simulink library "Lib_Piccolo"  (R2018b)
settings: Solver=VariableStepAuto  StartTime=0.0  StopTime=10.0  RelTol=1e-3
values from neighbouring files (symbols this model uses):
  AccelErrInt2Brakes = 0.15    [SimulationControlConfig16P.m]    (also in SimulationControlConfig16P_F0.m; SimulationControlConfig16P_F2.m; SimulationControlConfig16P_LEGACY.m; SimulationControlConfigTAILLESS.m = 0.2)
  AileronMax = 25    [SimulationControlConfig16P.m]    (also in SimulationControlConfig16P_F0.m; SimulationControlConfig16P_F2.m; SimulationControlConfig16P_LEGACY.m; SimulationControlConfigTAILLESS.m)
  AileronPower = 0.00268    [SimulationControlConfig16P.m]    (also in SimulationControlConfig16P_F0.m; SimulationControlConfig16P_F2.m; SimulationControlConfig16P_LEGACY.m; SimulationControlConfigTAILLESS.m = 0.002266)
  AileronSurfaceMax = 45    [SimulationControlConfig16P.m]    (also in SimulationControlConfig16P_F0.m; SimulationControlConfig16P_F2.m; SimulationControlConfig16P_LEGACY.m; SimulationControlConfigTAILLESS_CGAFT_F0.m = 25)
  AileronTrim = 0    [SimulationControlConfig16P.m]    (also in SimulationControlConfig16P_F0.m; SimulationControlConfig16P_F2.m; SimulationControlConfig16P_LEGACY.m; SimulationControlConfigTAILLESS.m)
  Alt = 1000 + TerrainHeight    [SimulationStateConfig.m]
  AltCruise_m = Alt * 0.3048    [SimulationControlConfig16P.m]    (also in SimulationControlConfig16P_F2.m; SimulationControlConfigTAILLESS.m = Alt/3.28084; SimulationControlConfigTAILLESS_CGAFT_F0.m = 640; SimulationControlConfigTAILLESS_CGFWD_F0.m = 640)
  AltitudeRate2PitchCmdIntegratorInit = 0.1    [SimulationControlPre.m]
  AltMax = 10000    [SimulationControlConfig16P.m]    (also in SimulationControlConfig16P_F0.m; SimulationControlConfig16P_F2.m; SimulationControlConfig16P_LEGACY.m; SimulationControlConfigTAILLESS.m)
  AltMaxAccel = 2.5    [SimulationControlConfig16P.m]    (also in SimulationControlConfig16P_F0.m = 2; SimulationControlConfig16P_F2.m = 2; SimulationControlConfig16P_LEGACY.m = 0.9; SimulationControlConfigTAILLESS.m = 2)
  AltMin = 0    [SimulationControlConfig16P.m]    (also in SimulationControlConfig16P_F0.m; SimulationControlConfig16P_F2.m; SimulationControlConfig16P_LEGACY.m; SimulationControlConfigTAILLESS.m)
  AltRateCmd2Pitch = 0.26    [SimulationControlConfig16P.m]    (also in SimulationControlConfig16P_F0.m = 0.35; SimulationControlConfig16P_F2.m = 0.35; SimulationControlConfig16P_LEGACY.m = 0.6; SimulationControlConfigTAILLESS.m = 0.9)
  AltRateError2Pitch = 0.34    [SimulationControlConfig16P.m]    (also in SimulationControlConfig16P_F0.m = 0.61; SimulationControlConfig16P_F2.m = 0.61; SimulationControlConfig16P_LEGACY.m = 0.4; SimulationControlConfigTAILLESS.m = 0.3)
  AltRateErrorInt2Pitch = 0.61    [SimulationControlConfig16P.m]    (also in SimulationControlConfig16P_F0.m = 0.28; SimulationControlConfig16P_F2.m = 0.28; SimulationControlConfig16P_LEGACY.m = 0.45; SimulationControlConfigTAILLESS.m = 0.15)
  AltRateLpfCutOff = 3    [SimulationControlConfig16P.m]    (also in SimulationControlConfig16P_F0.m; SimulationControlConfig16P_F2.m; SimulationControlConfig16P_LEGACY.m; SimulationControlConfigTAILLESS.m = 5)
  AutoNosegear2Rudder = 26    [SimulationControlConfig16P.m]    (also in SimulationControlConfig16P_F0.m; SimulationControlConfig16P_F2.m; SimulationControlConfig16P_LEGACY.m; SimulationControlConfigTAILLESS.m = 25.2)
  b = 5.54    [SimulationControlConfig16P.m]    (also in SimulationControlConfig16P_F0.m; SimulationControlConfig16P_F2.m; SimulationControlConfig16P_LEGACY.m; SimulationControlConfigTAILLESS.m = 2.37)
  Bank2AileronIntegratorInit = 0    [SimulationControlPre.m]
  BankMax_User = BankMax_User/180*pi    (= 0.610865238198)    [SimulationControlConfig16P.m]    (also in SimulationControlConfig16P_F0.m = 0.523598775598; SimulationControlConfig16P_F2.m = 0.523598775598; SimulationControlConfig16P_LEGACY.m = 0.523598775598; SimulationControlConfigTAILLESS.m = 0.558505360638)
  baseLegFlaps = 20    [SimulationControlConfig16P.m]    (also in SimulationControlConfig16P_F0.m; SimulationControlConfig16P_F2.m = 15; SimulationControlConfig16P_LEGACY.m = 0; SimulationControlConfigTAILLESS.m = 0)
  C = GeneticOpt.C    [SimulationCostFunction.m]
  c = Sw/b    (= 0.841696750903)    [SimulationControlConfig16P.m]    (also in SimulationControlConfig16P_F0.m; SimulationControlConfig16P_F2.m; SimulationControlConfig16P_LEGACY.m; SimulationControlConfigTAILLESS.m = 0.354008438819)
  cell2WheelFactorMG = 5.98    [SimulationSensorConfig16P_LEGACY.m]
  cell2WheelFactorNG = 1    [SimulationSensorConfig16P_LEGACY.m]
  cellSatMaxMG = 15000    [SimulationSensorConfig16P.m]    (also in SimulationSensorConfig16P_LEGACY.m; SimulationSensorConfigTAILLESS7P.m; SimulationSensorConfigUTAIL7P.m)
  cellSatMaxNG = 1000    [SimulationSensorConfig16P.m]    (also in SimulationSensorConfig16P_LEGACY.m; SimulationSensorConfigTAILLESS7P.m; SimulationSensorConfigUTAIL7P.m)
  cellSatMinMG = -15000    [SimulationSensorConfig16P.m]    (also in SimulationSensorConfig16P_LEGACY.m; SimulationSensorConfigTAILLESS7P.m; SimulationSensorConfigUTAIL7P.m)
  cellSatMinNG = -1000    [SimulationSensorConfig16P.m]    (also in SimulationSensorConfig16P_LEGACY.m; SimulationSensorConfigTAILLESS7P.m; SimulationSensorConfigUTAIL7P.m)
  CL_Limit = CL_Max    (= 0.54)    [SimulationControlConfig16P.m]    (also in SimulationControlConfig16P_F0.m; SimulationControlConfig16P_F2.m = 0.638; SimulationControlConfig16P_LEGACY.m; SimulationControlConfigTAILLESS.m = 0.525)
  CL_Max = 0.54    [SimulationControlConfig16P.m]    (also in SimulationControlConfig16P_F0.m; SimulationControlConfig16P_F2.m = 0.638; SimulationControlConfig16P_LEGACY.m; SimulationControlConfigTAILLESS.m = 0.525)
  CL_Max_Nom = 0.465    [SimulationControlConfig16P.m]    (also in SimulationControlConfig16P_F0.m; SimulationControlConfig16P_F2.m = 0.563; SimulationControlConfig16P_LEGACY.m; SimulationControlConfigTAILLESS.m = 0.39)
  CL_Min = 0    [SimulationControlConfig16P.m]    (also in SimulationControlConfig16P_F0.m; SimulationControlConfig16P_F2.m; SimulationControlConfig16P_LEGACY.m; SimulationControlConfigTAILLESS.m)
  ClimbMaxFraction = 0.35    [SimulationControlConfig16P.m]    (also in SimulationControlConfig16P_F0.m = 0.17; SimulationControlConfig16P_F2.m = 0.17; SimulationControlConfig16P_LEGACY.m = 0.24; SimulationControlConfigTAILLESS.m = 0.21)
  ClimboutMaxBank = 7.0    (= 7)    [SimulationControlConfig16P.m]    (also in SimulationControlConfig16P_F0.m; SimulationControlConfig16P_F2.m; SimulationControlConfig16P_LEGACY.m; SimulationControlConfigTAILLESS.m = 5)
  ClimboutTimer = 7.0    (= 7)    [SimulationControlConfig16P.m]    (also in SimulationControlConfig16P_F0.m; SimulationControlConfig16P_F2.m; SimulationControlConfig16P_LEGACY.m; SimulationControlConfigTAILLESS.m)
  dCl_per_dFlap = 0.005581818    [SimulationControlConfig16P.m]    (also in SimulationControlConfig16P_F0.m = 0; SimulationControlConfig16P_F2.m = 0.0065; SimulationControlConfig16P_LEGACY.m = 0; SimulationControlConfigTAILLESS.m = 0)
  DecelerationCmd = 3.1    [SimulationControlConfig16P.m]    (also in SimulationControlConfig16P_F0.m; SimulationControlConfig16P_F2.m; SimulationControlConfig16P_LEGACY.m; SimulationControlConfigTAILLESS.m = 0.1)
  DeRotateLogicEndTimer = abs((NoseDownLimit_Deg-1)/DeRotateRamp_Dps)    [SimulationControlConfig16P.m]    (also in SimulationControlConfig16P_F0.m; SimulationControlConfig16P_F2.m; SimulationControlConfig16P_LEGACY.m; SimulationControlConfigTAILLESS.m)
  DeRotateLogicHoldNoseUpTimer = 0.1    [SimulationControlConfig16P.m]    (also in SimulationControlConfig16P_F0.m; SimulationControlConfig16P_F2.m; SimulationControlConfig16P_LEGACY.m; SimulationControlConfigTAILLESS.m)
  DeRotateLogicTimerTimeout = 2    [SimulationControlConfig16P.m]    (also in SimulationControlConfig16P_F0.m; SimulationControlConfig16P_F2.m; SimulationControlConfig16P_LEGACY.m; SimulationControlConfigTAILLESS.m)
  DeRotateLowerCmdSaturation = 0    [SimulationControlConfig16P.m]    (also in SimulationControlConfig16P_F0.m; SimulationControlConfig16P_F2.m; SimulationControlConfig16P_LEGACY.m; SimulationControlConfigTAILLESS.m)
  DeRotateRamp_Dps = 3    [SimulationControlConfig16P.m]    (also in SimulationControlConfig16P_F0.m; SimulationControlConfig16P_F2.m; SimulationControlConfig16P_LEGACY.m; SimulationControlConfigTAILLESS.m = 8)
  DeRotateUpperCmdSaturation = 7    [SimulationControlConfig16P.m]    (also in SimulationControlConfig16P_F0.m; SimulationControlConfig16P_F2.m; SimulationControlConfig16P_LEGACY.m; SimulationControlConfigTAILLESS.m)
  DescentMaxFraction = 0.22    [SimulationControlConfig16P.m]    (also in SimulationControlConfig16P_F0.m = 0.2; SimulationControlConfig16P_F2.m = 0.2; SimulationControlConfig16P_LEGACY.m = 0.2; SimulationControlConfigTAILLESS.m = 0.17)
  DesktopSimTerrainOffset_m = 0.406    [SimulationAircraftConfig.m]
  downwindFlaps = 0    [SimulationControlConfig16P.m]    (also in SimulationControlConfig16P_F0.m; SimulationControlConfig16P_F2.m = 15; SimulationControlConfig16P_LEGACY.m; SimulationControlConfigTAILLESS.m)
  downwindSplitAil = 0    [SimulationControlConfig16P_F2.m]
  DP_init = 0.5*1.225*V_init^2    [SimulationControlConfig16P.m]    (also in SimulationControlConfig16P_F0.m; SimulationControlConfig16P_F2.m; SimulationControlConfig16P_LEGACY.m; SimulationControlConfigTAILLESS.m)
  dscNoiseMG = 1    [SimulationSensorConfig16P_LEGACY.m]
  dscNoiseNG = 0.25    [SimulationSensorConfig16P_LEGACY.m]
  DSCnumBits = 24    [SimulationSensorConfig16P.m]    (also in SimulationSensorConfig16P_LEGACY.m; SimulationSensorConfigTAILLESS7P.m; SimulationSensorConfigUTAIL7P.m)
  DSCRangeMaxMG = 15000    [SimulationSensorConfig16P.m]    (also in SimulationSensorConfig16P_LEGACY.m; SimulationSensorConfigTAILLESS7P.m; SimulationSensorConfigUTAIL7P.m)
  DSCRangeMaxNG = 1000    [SimulationSensorConfig16P.m]    (also in SimulationSensorConfig16P_LEGACY.m; SimulationSensorConfigTAILLESS7P.m; SimulationSensorConfigUTAIL7P.m)
  DSCRangeMinMG = -15000    [SimulationSensorConfig16P.m]    (also in SimulationSensorConfig16P_LEGACY.m; SimulationSensorConfigTAILLESS7P.m; SimulationSensorConfigUTAIL7P.m)
  DSCRangeMinNG = -1000    [SimulationSensorConfig16P.m]    (also in SimulationSensorConfig16P_LEGACY.m; SimulationSensorConfigTAILLESS7P.m; SimulationSensorConfigUTAIL7P.m)
  dt = DLLSim.dt    [SimulationTimeStep.m]    (also in SimulationTrim.m = 0.02)
  EarlyTouchdownThreshold = 3.0    (= 3)    [SimulationControlConfig16P.m]    (also in SimulationControlConfig16P_F0.m; SimulationControlConfig16P_F2.m; SimulationControlConfig16P_LEGACY.m; SimulationControlConfigTAILLESS.m)
  ElevatorDeflectionRate = 15    [SimulationControlConfig16P.m]    (also in SimulationControlConfig16P_F0.m; SimulationControlConfig16P_F2.m; SimulationControlConfig16P_LEGACY.m = 12; SimulationControlConfigTAILLESS.m = 5)
  ElevatorMax = 25    [SimulationControlConfig16P.m]    (also in SimulationControlConfig16P_F0.m; SimulationControlConfig16P_F2.m; SimulationControlConfig16P_LEGACY.m; SimulationControlConfigTAILLESS.m)
  ElevatorPower = -0.002209    [SimulationControlConfig16P.m]    (also in SimulationControlConfig16P_F0.m; SimulationControlConfig16P_F2.m; SimulationControlConfig16P_LEGACY.m; SimulationControlConfigTAILLESS.m = -0.002668)
  ElevatorTrim = -3.5    [SimulationControlConfig16P.m]    (also in SimulationControlConfig16P_F0.m; SimulationControlConfig16P_F2.m; SimulationControlConfig16P_LEGACY.m; SimulationControlConfigTAILLESS.m = -3)
  elevonBias = 0    [SimulationControlConfig16P.m]    (also in SimulationControlConfig16P_F0.m; SimulationControlConfig16P_F2.m; SimulationControlConfig16P_LEGACY.m; SimulationControlConfigTAILLESS.m)
  Enable_TAS_Protection = 0    [SimulationControlConfig16P.m]    (also in SimulationControlConfig16P_F0.m; SimulationControlConfig16P_F2.m; SimulationControlConfig16P_LEGACY.m; SimulationControlConfigTAILLESS.m)
  EnableCrossTrackAbort = 1    [SimulationControlConfig16P.m]    (also in SimulationControlConfigTAILLESS.m; SimulationControlConfigTAILLESS_CGAFT_F0.m; SimulationControlConfigTAILLESS_CGFWD_F0.m; SimulationControlConfigTAILLESS_CGFWD_F2.m)
  EnergyBandwidth = 0.04    [SimulationControlConfig16P.m]    (also in SimulationControlConfig16P_F0.m = 0.03; SimulationControlConfig16P_F2.m = 0.03; SimulationControlConfig16P_LEGACY.m = 0.02; SimulationControlConfigTAILLESS.m = 0.06)
  EngineLhFuelCut = 0    [SimulationAircraftConfig.m]
  EngineRhFuelCut = 0    [SimulationAircraftConfig.m]
  FastThrottleRate = 0.075    [SimulationControlConfig16P.m]    (also in SimulationControlConfig16P_F0.m = 0.05; SimulationControlConfig16P_F2.m = 0.05; SimulationControlConfig16P_LEGACY.m = 0.05; SimulationControlConfigTAILLESS.m = 0.1)
  FilterWarmUpTime = 2    [SimulationSensorConfig16P.m]    (also in SimulationSensorConfig16P_LEGACY.m; SimulationSensorConfigTAILLESS7P.m; SimulationSensorConfigUTAIL7P.m)
  finalApproachFlaps = 20    [SimulationControlConfig16P.m]    (also in SimulationControlConfig16P_F0.m; SimulationControlConfig16P_F2.m = 15; SimulationControlConfig16P_LEGACY.m = 0; SimulationControlConfigTAILLESS.m = 0)
  finalApproachSplitAil = 20    [SimulationControlConfig16P_F2.m]
  FinalDescentSlope_Deg = testPlans(testIndx).descentSlope    [SimulationControlConfig16P.m]    (also in SimulationControlConfig16P_F0.m; SimulationControlConfig16P_F2.m; SimulationControlConfig16P_LEGACY.m; SimulationControlConfigTAILLESS.m)
  flapMax = 0    [SimulationControlConfig16P.m]    (also in SimulationControlConfig16P_F0.m = 35; SimulationControlConfig16P_F2.m = 33; SimulationControlConfig16P_LEGACY.m; SimulationControlConfigTAILLESS.m)
  flapRate = 7.5    [SimulationControlConfig16P.m]    (also in SimulationControlConfig16P_F0.m; SimulationControlConfig16P_F2.m; SimulationControlConfig16P_LEGACY.m; SimulationControlConfigTAILLESS.m = 6.6)
  FlareHeight = 5    [SimulationControlConfig16P.m]    (also in SimulationControlConfig16P_F0.m; SimulationControlConfig16P_F2.m; SimulationControlConfig16P_LEGACY.m = 4.8; SimulationControlConfigTAILLESS.m = 2.75)
  FlareVerticalRate_mps = -0.4    [SimulationControlConfig16P.m]    (also in SimulationControlConfig16P_F0.m; SimulationControlConfig16P_F2.m; SimulationControlConfig16P_LEGACY.m = -0.5; SimulationControlConfigTAILLESS.m = -0.15)
  Fp_Aileron = 0.55*2*pi*RollRateLpfCutoff*dt    [SimulationControlConfig16P.m]    (also in SimulationControlConfig16P_F0.m; SimulationControlConfig16P_F2.m; SimulationControlConfig16P_LEGACY.m; SimulationControlConfigTAILLESS.m)
  Fp_Alt = 2*pi*0.55*AltBandwidth    (= 0.622035345411)    [SimulationControlConfig16P.m]    (also in SimulationControlConfig16P_F0.m; SimulationControlConfig16P_F2.m; SimulationControlConfig16P_LEGACY.m = 0.099; SimulationControlConfigTAILLESS.m = 0.207345115137)
  Fp_AltRate = 0.55*2*pi*AltRateLpfCutOff*dt    [SimulationControlConfig16P.m]    (also in SimulationControlConfig16P_F0.m; SimulationControlConfig16P_F2.m; SimulationControlConfig16P_LEGACY.m; SimulationControlConfigTAILLESS.m)
  Fp_Elevator = 0.55*2*pi*PitchRateLpfCutoff*dt    [SimulationControlConfig16P.m]    (also in SimulationControlConfig16P_F0.m; SimulationControlConfig16P_F2.m; SimulationControlConfig16P_LEGACY.m; SimulationControlConfigTAILLESS.m)
  Fp_Energy = 0.55*2*pi*EnergyBandwidth    (= 0.138230076758)    [SimulationControlConfig16P.m]    (also in SimulationControlConfig16P_F0.m = 0.103672557568; SimulationControlConfig16P_F2.m = 0.103672557568; SimulationControlConfig16P_LEGACY.m = 0.069115038379; SimulationControlConfigTAILLESS.m = 0.207345115137)
  Fp_Energy2 = 0.55*2*pi*EnergyBandwidth*dt    [SimulationControlConfig16P.m]    (also in SimulationControlConfig16P_F0.m; SimulationControlConfig16P_F2.m; SimulationControlConfig16P_LEGACY.m; SimulationControlConfigTAILLESS.m)
  Fp_Pitch = 0.55*2*pi*PitchBandwidth    (= 2.45358386245)    [SimulationControlConfig16P.m]    (also in SimulationControlConfig16P_F0.m; SimulationControlConfig16P_F2.m = 1.72787595947; SimulationControlConfig16P_LEGACY.m = 3.11017672705; SimulationControlConfigTAILLESS.m = 1.55508836353)
  Fp_Pitch_2 = 0.55*2*pi*PitchBandwidth*dt    [SimulationControlConfig16P.m]    (also in SimulationControlConfig16P_F0.m; SimulationControlConfig16P_F2.m; SimulationControlConfig16P_LEGACY.m; SimulationControlConfigTAILLESS.m)
  Fp_Roll = RollBandwidth^2    (= 1.69)    [SimulationControlConfig16P.m]    (also in SimulationControlConfig16P_F0.m = 1.44; SimulationControlConfig16P_F2.m = 1.44; SimulationControlConfig16P_LEGACY.m = 1.44; SimulationControlConfigTAILLESS.m = 1.21)
  Fp_Rudder = 0.55*2*pi*YawRateLpfCutoff*dt    [SimulationControlConfig16P.m]    (also in SimulationControlConfig16P_F0.m; SimulationControlConfig16P_F2.m; SimulationControlConfig16P_LEGACY.m; SimulationControlConfigTAILLESS.m)
  Fp_TAS = 0.55*2*pi*TASBandwidth    (= 0.103672557568)    [SimulationControlConfig16P.m]    (also in SimulationControlConfig16P_F0.m; SimulationControlConfig16P_F2.m; SimulationControlConfig16P_LEGACY.m; SimulationControlConfigTAILLESS.m = 0.172787595947)
  Fp_TAS_Filter = 2*pi*TasLpfCutoff*dt    [SimulationControlConfig16P.m]    (also in SimulationControlConfig16P_F0.m; SimulationControlConfig16P_F2.m; SimulationControlConfig16P_LEGACY.m; SimulationControlConfigTAILLESS.m)
  Fp_Turn = 0.55*2*pi*TurnErrLPFcutoff    (= 0.172787595947)    [SimulationControlConfig16P.m]    (also in SimulationControlConfig16P_F0.m = 0.0345575191895; SimulationControlConfig16P_F2.m = 0.0345575191895; SimulationControlConfig16P_LEGACY.m = 0.0345575191895; SimulationControlConfigTAILLESS.m)
  Fp_TurnDerr = 0.55*2*pi*TurnDerivativeLPFcutoff    (= 0.172787595947)    [SimulationControlConfig16P.m]    (also in SimulationControlConfig16P_F0.m = 0.0345575191895; SimulationControlConfig16P_F2.m = 0.0345575191895; SimulationControlConfig16P_LEGACY.m = 0.0345575191895; SimulationControlConfigTAILLESS.m)
  FTV = 3    [SimulationAircraftConfig.m]
  ftvStaticPositionError = 1/1.18    (= 0.847457627119)    [SimulationSensorConfig16P.m]    (also in SimulationSensorConfig16P_LEGACY.m; SimulationSensorConfigTAILLESS7P.m = 1; SimulationSensorConfigUTAIL7P.m = 1)
  g = 9.81    [SimulationStateConfig.m]
  goAroundSplitAil = 0    [SimulationControlConfig16P_F2.m]
  GustSpd_Kts = testPlans(testIndx).gustSpd    [SimulationStateConfig.m]
  GustTriggerVal = testPlans(testIndx).gustTriggerVal    [SimulationStateConfig.m]
  HeadingErr2TurnRate = 0.5    [SimulationControlConfig16P.m]    (also in SimulationControlConfig16P_F0.m; SimulationControlConfig16P_F2.m; SimulationControlConfig16P_LEGACY.m; SimulationControlConfigTAILLESS.m)
  HeadingErrDer2TurnRate = 0.3    [SimulationControlConfig16P.m]    (also in SimulationControlConfig16P_F0.m; SimulationControlConfig16P_F2.m; SimulationControlConfig16P_LEGACY.m; SimulationControlConfigTAILLESS.m)
  IASbounce = IASstall*0.8    [SimulationControlPre.m]
  IAScruiseCMD = sqrt(2*m*9.81/(1.225*Sw*CL_cruise))    [SimulationControlConfig16P.m]    (also in SimulationControlConfig16P_F0.m; SimulationControlConfig16P_F2.m; SimulationControlConfig16P_LEGACY.m; SimulationControlConfigTAILLESS.m)
  IASfinalCMD = 1.12 * IASmin    [SimulationControlConfig16P.m]    (also in SimulationControlConfig16P_F0.m = 1.14 * IASmin; SimulationControlConfig16P_F2.m = 1.10 * IASmin; SimulationControlConfig16P_LEGACY.m = 1.10 * IASmin; SimulationControlConfigTAILLESS.m = 1.14 * IASmin)
  IASflareCMD = IASstall    [SimulationControlConfig16P.m]    (also in SimulationControlConfig16P_F0.m; SimulationControlConfig16P_F2.m; SimulationControlConfig16P_LEGACY.m; SimulationControlConfigTAILLESS.m)
  IASmax = 64    [SimulationControlConfig16P.m]    (also in SimulationControlConfig16P_F0.m = 46; SimulationControlConfig16P_F2.m = 52; SimulationControlConfig16P_LEGACY.m = 46; SimulationControlConfigTAILLESS.m = 38.9)
  IASmin = sqrt(2*m*9.81/(1.225*Sw*0.9*CL_Max_Nom))    [SimulationControlConfig16P.m]    (also in SimulationControlConfig16P_F0.m; SimulationControlConfig16P_F2.m; SimulationControlConfig16P_LEGACY.m; SimulationControlConfigTAILLESS.m)
  IASshortCMD = IASstall    [SimulationControlConfig16P.m]    (also in SimulationControlConfig16P_F0.m; SimulationControlConfig16P_F2.m; SimulationControlConfig16P_LEGACY.m; SimulationControlConfigTAILLESS.m)
  IASstall = sqrt(2*m*9.81/(1.225*Sw*CL_Max))    [SimulationControlConfig16P.m]    (also in SimulationControlConfig16P_F0.m; SimulationControlConfig16P_F2.m; SimulationControlConfig16P_LEGACY.m; SimulationControlConfigTAILLESS.m)
  inFlight = 1    [SimulationControlConfig16P.m]    (also in SimulationControlConfigTAILLESS.m; SimulationControlConfigTAILLESS_CGAFT_F0.m; SimulationControlConfigTAILLESS_CGFWD_F0.m; SimulationControlConfigTAILLESS_CGFWD_F2.m)
  JetCatOffset = 5    [SimulationControlConfig16P.m]    (also in SimulationControlConfig16P_F0.m; SimulationControlConfig16P_F2.m; SimulationControlConfig16P_LEGACY.m)
  LaunchRollingElevator = -1.5    [SimulationControlConfig16P.m]    (also in SimulationControlConfig16P_F0.m; SimulationControlConfig16P_F2.m = 1.25; SimulationControlConfig16P_LEGACY.m; SimulationControlConfigTAILLESS.m = 1)
  ldg_NosegearMax = 10    [SimulationControlConfig16P.m]    (also in SimulationControlConfig16P_F0.m; SimulationControlConfig16P_F2.m; SimulationControlConfig16P_LEGACY.m; SimulationControlConfigTAILLESS.m)
  ldg_TrackVyErrInt2Nosegear = 0.1250    (= 0.125)    [SimulationControlConfig16P.m]    (also in SimulationControlConfig16P_F0.m; SimulationControlConfig16P_F2.m; SimulationControlConfig16P_LEGACY.m; SimulationControlConfigTAILLESS.m = 0.00714285714286)
  ldg_TrackVyErrPro2Nosegear = 0.35    [SimulationControlConfig16P.m]    (also in SimulationControlConfig16P_F0.m; SimulationControlConfig16P_F2.m; SimulationControlConfig16P_LEGACY.m; SimulationControlConfigTAILLESS.m = 0.0546666666667)
  ldg_TrackY2Vy = 0.07    [SimulationControlConfig16P.m]    (also in SimulationControlConfig16P_F0.m; SimulationControlConfig16P_F2.m; SimulationControlConfig16P_LEGACY.m; SimulationControlConfigTAILLESS.m = 0.17)
  ldg_Vy2NosegearScalingPower = 1.075    [SimulationControlConfig16P.m]    (also in SimulationControlConfig16P_F0.m; SimulationControlConfig16P_F2.m; SimulationControlConfig16P_LEGACY.m; SimulationControlConfigTAILLESS.m = 0.6)
  ldg_Y2VyScalingPower = 0.175    [SimulationControlConfig16P.m]    (also in SimulationControlConfig16P_F0.m; SimulationControlConfig16P_F2.m; SimulationControlConfig16P_LEGACY.m; SimulationControlConfigTAILLESS.m = 0)
  ldg_YawRate2Nosegear = 0.175    [SimulationControlConfig16P.m]    (also in SimulationControlConfig16P_F0.m; SimulationControlConfig16P_F2.m; SimulationControlConfig16P_LEGACY.m; SimulationControlConfigTAILLESS.m = 0.065)
  LiftSlope = 0.064285    [SimulationControlConfig16P.m]    (also in SimulationControlConfig16P_F0.m; SimulationControlConfig16P_F2.m; SimulationControlConfig16P_LEGACY.m; SimulationControlConfigTAILLESS.m = 0.058631)
  LPFaileronInit = 0    [SimulationControlPre.m]
  LPFclestInit = 0    [SimulationControlPre.m]
  LPFenergyFFInit = 0    [SimulationControlPre.m]
  ... (+122 more)
undefined symbols (not defined in the file or in its folder): abortFlag, alphaHPF, apmDelay, BRWNOUT, CRAWOR, CRAWUR, DiscIntNeverNeededParam, DLLSim, DLLSimStep, ECOMOR, ECOMUR, Fp_Tas, GustTrigger_HeightAgl_m, IPSTAT, LCINTEG, Ldg_Persist_Time, LOWER_FLAGS, MSG_ENABLE, NoiseStd, OLDVAL, OVERRIDE_ENABLE, OVERRIDE_VALUE, REBOOT, reversionEnable, revIASMax, revIASMin, revPitchMax, revPitchMin, revPitchRateMax, revRollMax, revRollRateMax, SAMPLE, SCALON, SensorModel, sigbuilder_block, Sim_Vx, Sim_Vy, Sim_Vz, Sim_Xpos, Sim_Ypos, Sim_Zpos, SYSOR, SYSUR, TARE, TEMPOR, TEMPUR, testIndx, testPlan, testPlans, Trim_piccoloInCmd, Trim_REFSI_FD_IN_nmodeCgShifterCmd_Flag, Trim_REFSI_FD_IN_nmodeCgShifterCmd_Ft, Trim_REFSI_FD_IN_nmodeCgShifterCmdType, Trim_REFSI_FD_IN_nmodeCgShifterNRCActive, Trim_REFSI_FD_IN_nmodeFlapLhIBCmd_Deg, Trim_REFSI_FD_IN_nmodeFlapLhOBCmd_Deg, Trim_REFSI_FD_IN_nmodeFlapRhIBCmd_Deg, Trim_REFSI_FD_IN_nmodeFlapRhOBCmd_Deg, Trim_REFSI_FD_IN_nmodeSlatLhCmd_Deg ... (+11)
libraries: simulink x1237, $bdroot x179, aerolibconvert2 x63, dspswit3 x25, aerolibatmos2 x5, simulink_extras x4, dsparch4 x2, Lib_Piccolo_Alt x2, eeGeneralControl x1, dspindex x1
(part 22 of 74)

== system Lib_Piccolo/A//C Dynamics Full Interface/Simulated Piccolo Commands/16P5 ==
  Aileron : Inport
  Inboard Elevon : Inport  Port=2
  Outboard Elevon : Inport  Port=3
  U-Tail Elevator : Inport  Port=4
  Aft-Flap : Inport  Port=5
  "PylonRudder " : Inport  Port=6
  "WingletRudder " : Inport  Port=7
  U-Tail Rudder : Inport  Port=8
  "Throttle " : Inport  Port=9
  Nosegear : Inport  Port=10
  Flaps : Inport  Port=11
  Slats : Inport  Port=12
  Spoilers : Inport  Port=13
  Brake : Inport  Port=14
  Stabilizer : Inport  Port=15
  CG_Shifter : Inport  Port=16
  Add : Sum  Commented=on  Inputs=|++
  Bus Selector : BusSelector  OutputSignals=PrtAileronUpperCmd_Deg,PrtAileronLowerCmd_Deg,StbdAileronUpperCmd_Deg,StbdAileronLowerCmd_Deg
  Bus Selector1 : BusSelector  OutputSignals=PrtOutElevonCmd_Deg,StbdOutElevonCmd_Deg
  Bus Selector2 : BusSelector  OutputSignals=PrtThrottleCmd_Pct,StbdThrottleCmd_Pct
  Bus Selector3 : BusSelector  OutputSignals=PrtInbElevonCmd_Deg,StbdInbElevonCmd_Deg
  Bus Selector4 : BusSelector  OutputSignals=StabLhCmdDeg
  Constant : Constant  Value=0
  Constant1 : Constant  Value=0
  Constant2 : Constant  Value=0
  Constant3 : Constant
  Constant4 : Constant  Value=Trim_REFSI_FD_IN_nmodeCgShifterCmd_Flag
  Constant5 : Constant  Value=Trim_REFSI_FD_IN_nmodeCgShifterNRCActive
  Gain{,1..20} (21 alike) : Gain
  Goto Tag Visibility1 : GotoTagVisibility  GotoTag=CLAWsOn
  Signal Builder2 : Subsystem  Tag=STV Subsys  Commented=on  LoadFcn=sigbuilder_block('load');  StartFcn=sigbuilder_block('start');  StopFcn=sigbuilder_block('stop');  ClipboardFcn=sigbuilder_block('clipboard');  mask(Sigbuilder block){tuvar=[0:10]}
      mask help: Simulink:masks:SigbuilderBlock_MD
      mask init:
      | if ~strcmp(get_param(bdroot(gcbh),'SimulationStatus'),'stopped') tuvar = sigbuilder_block('maskInit'); end
      settings: CopyFcn=sigbuilder_block('copy');  DeleteFcn=sigbuilder_block('delete');  ModelCloseFcn=sigbuilder_block('modelClose');  PreSaveFcn=sigbuilder_block('preSave');  PauseFcn=sigbuilder_block('pause');  ContinueFcn=sigbuilder_block('continue');  NameChangeFcn=sigbuilder_block('namechange');  OpenFcn=sigbuilder_block('open',[421.8 380.4 544.2 313.2 ]);  CloseFcn=sigbuilder_block('close');
      mask Display: plot(0, 0, 100, 100,[2, 2, 32, 32, 2], [68, 8, 8, 68, 68],[32, 2], [38, 38], [32, 19, 2],[53, 60, 44], [32, 17, 17, 2],[16, 16, 31, 31]);txt = getActiveGroup(gcbh);text(2, 100, txt,'verticalAlignment', 'top');
  SimInputBusCreator : BusCreator  Inputs=46
  Subsystem : Subsystem
  Subsystem1 : Subsystem
  Subsystem10 : Subsystem
  Subsystem11 : Subsystem
  Subsystem12 : Subsystem
  Subsystem13 : Subsystem
  Subsystem14 : Subsystem
  Subsystem15 : Subsystem
  Subsystem16 : Subsystem
  Subsystem2 : Subsystem
  Subsystem3 : Subsystem
  Subsystem4 : Subsystem
  Subsystem5 : Subsystem
  Subsystem6 : Subsystem
  Subsystem7 : Subsystem
  Subsystem8 : Subsystem
  Subsystem9 : Subsystem
  nmodeTlaRhCmdDeg1 : Constant  Commented=on  Value=Trim_piccoloInCmd
  nmodeTlaRhCmdDeg2 : Constant  Value=0
  nmodeTlaRhCmdDeg3 : Constant  Value=EngineLhFuelCut
  nmodeTlaRhCmdDeg4 : Constant  Value=WindDir_Deg
  nmodeTlaRhCmdDeg5 : Constant  Value=EngineRhFuelCut
  nmodeTlaRhCmdDeg6 : Constant  Value=WindSpd_Kts
  nmodeTlaRhCmdDeg7 : Constant  Value=WindVertSpd_Kts
  unity35 : Gain
  unity36 : Gain
  Command Bundle : Outport
  tag scope: CLAWsOn=scoped
  wires:
  Stabilizer/1 -> Bus Selector4/1
  nmodeTlaRhCmdDeg7/1 -> SimInputBusCreator/42  "VertWindSpdKts"
  Gain20/1 -> SimInputBusCreator/18  "REFSI_FD_IN_nmodeStabCmd"
  Subsystem4/1(CLAWS_ElvLhIBCmdDeg) -> SimInputBusCreator/5
  Subsystem/1(CLAWS_RudWingletLhCmdDeg) -> SimInputBusCreator/1
  nmodeTlaRhCmdDeg3/1 -> SimInputBusCreator/27  "EngineLhFuelCut"
  Subsystem2/1(CLAWS_AilUprLhCmdDeg) -> SimInputBusCreator/3
  Gain15/1 -> SimInputBusCreator/22  "REFSI_FD_IN_nmodeSlatRhPosn_Deg"
  Gain14/1 -> SimInputBusCreator/21  "REFSI_FD_IN_nmodeSlatLhPosn_Deg"
  Subsystem10/1(CLAWS_RudUTailRhCmdDeg) -> SimInputBusCreator/11
  Subsystem14/1(CLAWS_AilUprRhCmdDeg) -> SimInputBusCreator/15
  Subsystem6/1(CLAWS_RudUTailLhCmdDeg) -> SimInputBusCreator/7
  Subsystem5/1(CLAWS_RudPylLhCmdDeg) -> SimInputBusCreator/6
  Subsystem8/1(CLAWS_AftFlapCmdDeg) -> SimInputBusCreator/9
  Nosegear/1 -> SimInputBusCreator/30  "REFSI_FD_IN_nmodeNoseGearCmd_Deg"
  Subsystem12/1(CLAWS_ElvRhIBCmdDeg) -> SimInputBusCreator/13
  Subsystem16/1(CLAWS_RudWingletRhCmdDeg) -> SimInputBusCreator/17
  Gain10/1 -> SimInputBusCreator/31  "REFSI_FD_IN_nmodeSplrLhOutbdCmd_Deg"
  nmodeTlaRhCmdDeg2/1 -> [CLAWsOn]
  Subsystem13/1(CLAWS_ElvRhOBCmdDeg) -> SimInputBusCreator/14
  Aft-Flap/1 -> Subsystem8/1(In1)
  Signal Builder2/1(Signal 3) -> Add/2
  nmodeTlaRhCmdDeg1/1 -> Add/1
  Subsystem11/1(CLAWS_RudPylRhCmdDeg) -> SimInputBusCreator/12
  "PylonRudder "/1 -> Subsystem11/1(In1), Subsystem5/1(In1)
  Gain18/1 -> SimInputBusCreator/23  "REFSI_FD_IN_nmodeFlapRhOBPosn_Deg"
  Subsystem9/1(CLAWS_ElvUTailRhCmdDeg) -> SimInputBusCreator/10
  Gain13/1 -> SimInputBusCreator/34  "REFSI_FD_IN_nmodeSplrRhOutbdCmd_Deg"
  nmodeTlaRhCmdDeg5/1 -> SimInputBusCreator/28  "EngineRhFuelCut"
  Gain17/1 -> SimInputBusCreator/20  "REFSI_FD_IN_nmodeFlapLhIBPosn_Deg"
  U-Tail Rudder/1 -> Subsystem10/1(In1), Subsystem6/1(In1)
  Gain19/1 -> SimInputBusCreator/24  "REFSI_FD_IN_nmodeFlapRhIBPosn_Deg"
  Gain16/1 -> SimInputBusCreator/19  "REFSI_FD_IN_nmodeFlapLhOBPosn_Deg"
  Subsystem1/1(CLAWS_AilLwrLhCmdDeg) -> SimInputBusCreator/2
  "WingletRudder "/1 -> Subsystem/1(In1), Subsystem16/1(In1)
  Subsystem3/1(CLAWS_ElvLhOBCmdDeg) -> SimInputBusCreator/4
  Subsystem7/1(CLAWS_ElvUTailLhCmdDeg) -> SimInputBusCreator/8
  Gain12/1 -> SimInputBusCreator/33  "REFSI_FD_IN_nmodeSplrRhInbdCmd_Deg"
  Subsystem15/1(CLAWS_AilLwrRhCmdDeg) -> SimInputBusCreator/16
  CG_Shifter/1 -> SimInputBusCreator/35  "REFSI_FD_IN_nmodeCgShifterCmd_Ft"
  Gain11/1 -> SimInputBusCreator/32  "REFSI_FD_IN_nmodeSplrLhInbdCmd_Deg"
  Brake/1 -> unity36/1, unity35/1, SimInputBusCreator/29  "REFSI_FD_IN_nmodeBrakeCmd"
  U-Tail Elevator/1 -> Subsystem9/1(In1), Subsystem7/1(In1)
  SimInputBusCreator/1 -> Command Bundle/1
  Gain/1 -> Subsystem14/1(In1)
  Gain1/1 -> Subsystem15/1(In1)
  Gain2/1 -> Subsystem12/1(In1)
  Gain3/1 -> Subsystem13/1(In1)
  Gain4/1 -> Subsystem1/1(In1)
  Gain5/1 -> Subsystem2/1(In1)
  Gain6/1 -> Subsystem3/1(In1)
  Gain7/1 -> Subsystem4/1(In1)
  Constant1/1 -> SimInputBusCreator/37  "pilotNzCmd_g"
  Constant/1 -> SimInputBusCreator/36  "piccoloInCmd"
  Constant2/1 -> SimInputBusCreator/38  "isControlSurfaceCmdFromSystem"
  Constant3/1 -> SimInputBusCreator/39  "nmodeReset"
  nmodeTlaRhCmdDeg4/1 -> SimInputBusCreator/40  "RefWindDirDeg"
  nmodeTlaRhCmdDeg6/1 -> SimInputBusCreator/41  "RefWindSpdKts"
  unity36/1 -> SimInputBusCreator/44  "PedalBrakeRh"
  unity35/1 -> SimInputBusCreator/43  "PedalBrakeLh"
  Gain8/1 -> SimInputBusCreator/25  "REFSI_FD_IN_nmodeTlaLhCmd_Deg"
  Gain9/1 -> SimInputBusCreator/26  "REFSI_FD_IN_nmodeTlaRhCmd_Deg"
  Aileron/1 -> Bus Selector/1
  Bus Selector/1 -> Gain4/1  "<PrtAileronUpperCmd_Deg>"
  Bus Selector/2 -> Gain5/1  "<PrtAileronLowerCmd_Deg>"
  Bus Selector/3 -> Gain/1  "<StbdAileronUpperCmd_Deg>"
  Bus Selector/4 -> Gain1/1  "<StbdAileronLowerCmd_Deg>"
  Outboard Elevon/1 -> Bus Selector1/1
  Bus Selector1/1 -> Gain6/1  "<PrtOutElevonCmd_Deg>"
  Bus Selector1/2 -> Gain3/1  "<StbdOutElevonCmd_Deg>"
  "Throttle "/1 -> Bus Selector2/1
  Bus Selector2/1 -> Gain8/1  "<PrtThrottleCmd_Pct>"
  Bus Selector2/2 -> Gain9/1  "<StbdThrottleCmd_Pct>"
  Inboard Elevon/1 -> Bus Selector3/1
  Bus Selector3/1 -> Gain7/1  "<PrtInbElevonCmd_Deg>"
  Bus Selector3/2 -> Gain2/1  "<StbdInbElevonCmd_Deg>"
  Spoilers/1 -> Gain13/1, Gain12/1, Gain11/1, Gain10/1
  Slats/1 -> Gain15/1, Gain14/1
  Flaps/1 -> Gain19/1, Gain18/1, Gain17/1, Gain16/1
  Bus Selector4/1 -> Gain20/1  "<StabLhCmdDeg>"
  Constant4/1 -> SimInputBusCreator/45  "REFSI_FD_IN_nmodeCgShifterCmd_Flag"
  Constant5/1 -> SimInputBusCreator/46  "REFSI_FD_IN_nmodeCgShifterNRCActive"

== system Lib_Piccolo/A//C Dynamics Full Interface/Simulated Piccolo Commands/16P5_DualHStab ==
  Aileron : Inport
  Inboard Elevon : Inport  Port=2
  Outboard Elevon : Inport  Port=3
  U-Tail Elevator : Inport  Port=4
  Aft-Flap : Inport  Port=5
  "PylonRudder " : Inport  Port=6
  "WingletRudder " : Inport  Port=7
  U-Tail Rudder : Inport  Port=8
  "Throttle " : Inport  Port=9
  Nosegear : Inport  Port=10
  Brake : Inport  Port=11
  Flaps : Inport  Port=12
  Slats : Inport  Port=13
  Spoilers : Inport  Port=14
  Stabilizer : Inport  Port=15
  CG_Shifter : Inport  Port=16
  Add : Sum  Commented=on  Inputs=|++
  Bus Selector : BusSelector  OutputSignals=PrtAileronUpperCmd_Deg,PrtAileronLowerCmd_Deg,StbdAileronUpperCmd_Deg,StbdAileronLowerCmd_Deg
  Bus Selector1 : BusSelector  OutputSignals=PrtOutElevonCmd_Deg,StbdOutElevonCmd_Deg
  Bus Selector2 : BusSelector  OutputSignals=PrtThrottleCmd_Pct,StbdThrottleCmd_Pct
  Bus Selector3 : BusSelector  OutputSignals=PrtInbElevonCmd_Deg,StbdInbElevonCmd_Deg
  Bus Selector4 : BusSelector  OutputSignals=StabLhCmdDeg,StabRhCmdDeg
  Constant : Constant  Value=0
  Constant1 : Constant  Value=0
  Constant2 : Constant  Value=0
  Constant3 : Constant
  Constant4 : Constant  Value=Trim_REFSI_FD_IN_nmodeCgShifterCmdType
  Constant5 : Constant  Commented=on  Value=Trim_REFSI_FD_IN_nmodeCgShifterNRCActive
  Constant6 : Constant
  Gain{,1..21} (22 alike) : Gain
  Goto Tag Visibility1 : GotoTagVisibility  GotoTag=CLAWsOn
  Signal Builder2 : Subsystem  Tag=STV Subsys  Commented=on  LoadFcn=sigbuilder_block('load');  StartFcn=sigbuilder_block('start');  StopFcn=sigbuilder_block('stop');  ClipboardFcn=sigbuilder_block('clipboard');  mask(Sigbuilder block){tuvar=[0:10]}
      mask help: Simulink:masks:SigbuilderBlock_MD
      mask init:
      | if ~strcmp(get_param(bdroot(gcbh),'SimulationStatus'),'stopped') tuvar = sigbuilder_block('maskInit'); end
      settings: CopyFcn=sigbuilder_block('copy');  DeleteFcn=sigbuilder_block('delete');  ModelCloseFcn=sigbuilder_block('modelClose');  PreSaveFcn=sigbuilder_block('preSave');  PauseFcn=sigbuilder_block('pause');  ContinueFcn=sigbuilder_block('continue');  NameChangeFcn=sigbuilder_block('namechange');  OpenFcn=sigbuilder_block('open',[421.8 380.4 544.2 313.2 ]);  CloseFcn=sigbuilder_block('close');
      mask Display: plot(0, 0, 100, 100,[2, 2, 32, 32, 2], [68, 8, 8, 68, 68],[32, 2], [38, 38], [32, 19, 2],[53, 60, 44], [32, 17, 17, 2],[16, 16, 31, 31]);txt = getActiveGroup(gcbh);text(2, 100, txt,'verticalAlignment', 'top');
  SimInputBusCreator : BusCreator  Inputs=47
  Subsystem : Subsystem
  Subsystem1 : Subsystem
  Subsystem10 : Subsystem
  Subsystem11 : Subsystem
  Subsystem12 : Subsystem
  Subsystem13 : Subsystem
  Subsystem14 : Subsystem
  Subsystem15 : Subsystem
  Subsystem16 : Subsystem
  Subsystem2 : Subsystem
  Subsystem3 : Subsystem
  Subsystem4 : Subsystem
  Subsystem5 : Subsystem
  Subsystem6 : Subsystem
  Subsystem7 : Subsystem
  Subsystem8 : Subsystem
  Subsystem9 : Subsystem
  nmodeTlaRhCmdDeg1 : Constant  Commented=on  Value=Trim_piccoloInCmd
  nmodeTlaRhCmdDeg2 : Constant  Value=0
  nmodeTlaRhCmdDeg3 : Constant  Value=EngineLhFuelCut
  nmodeTlaRhCmdDeg4 : Constant  Value=WindDir_Deg
  nmodeTlaRhCmdDeg5 : Constant  Value=EngineRhFuelCut
  nmodeTlaRhCmdDeg6 : Constant  Value=WindSpd_Kts
  nmodeTlaRhCmdDeg7 : Constant  Value=WindVertSpd_Kts
  unity35 : Gain
  unity36 : Gain
  Command Bundle : Outport
  tag scope: CLAWsOn=scoped
  wires:
  Bus Selector4/1 -> Gain21/1  "<StabLhCmdDeg>"
  Gain21/1 -> SimInputBusCreator/18  "REFSI_FD_IN_nmodeStabLhCmd"
  Stabilizer/1 -> Bus Selector4/1
  Bus Selector4/2 -> Gain20/1  "<StabRhCmdDeg>"
  nmodeTlaRhCmdDeg7/1 -> SimInputBusCreator/43  "VertWindSpdKts"
  Gain20/1 -> SimInputBusCreator/19  "REFSI_FD_IN_nmodeStabRhCmd"
  Subsystem4/1(CLAWS_ElvLhIBCmdDeg) -> SimInputBusCreator/5
  Subsystem/1(CLAWS_RudWingletLhCmdDeg) -> SimInputBusCreator/1
  nmodeTlaRhCmdDeg3/1 -> SimInputBusCreator/28  "EngineLhFuelCut"
  Subsystem2/1(CLAWS_AilUprLhCmdDeg) -> SimInputBusCreator/3
  Gain15/1 -> SimInputBusCreator/23  "REFSI_FD_IN_nmodeSlatRhPosn_Deg"
  Gain14/1 -> SimInputBusCreator/22  "REFSI_FD_IN_nmodeSlatLhPosn_Deg"
  Subsystem10/1(CLAWS_RudUTailRhCmdDeg) -> SimInputBusCreator/11
  Subsystem14/1(CLAWS_AilUprRhCmdDeg) -> SimInputBusCreator/15
  Subsystem6/1(CLAWS_RudUTailLhCmdDeg) -> SimInputBusCreator/7
  Subsystem5/1(CLAWS_RudPylLhCmdDeg) -> SimInputBusCreator/6
  Subsystem8/1(CLAWS_AftFlapCmdDeg) -> SimInputBusCreator/9
  Nosegear/1 -> SimInputBusCreator/31  "REFSI_FD_IN_nmodeNoseGearCmd_Deg"
  Subsystem12/1(CLAWS_ElvRhIBCmdDeg) -> SimInputBusCreator/13
  Subsystem16/1(CLAWS_RudWingletRhCmdDeg) -> SimInputBusCreator/17
  Gain10/1 -> SimInputBusCreator/32  "REFSI_FD_IN_nmodeSplrLhOutbdCmd_Deg"
  nmodeTlaRhCmdDeg2/1 -> [CLAWsOn]
  Subsystem13/1(CLAWS_ElvRhOBCmdDeg) -> SimInputBusCreator/14
  Aft-Flap/1 -> Subsystem8/1(In1)
  Signal Builder2/1(Signal 3) -> Add/2
  nmodeTlaRhCmdDeg1/1 -> Add/1
  Subsystem11/1(CLAWS_RudPylRhCmdDeg) -> SimInputBusCreator/12
  "PylonRudder "/1 -> Subsystem11/1(In1), Subsystem5/1(In1)
  Gain18/1 -> SimInputBusCreator/24  "REFSI_FD_IN_nmodeFlapRhOBPosn_Deg"
  Subsystem9/1(CLAWS_ElvUTailRhCmdDeg) -> SimInputBusCreator/10
  Gain13/1 -> SimInputBusCreator/35  "REFSI_FD_IN_nmodeSplrRhOutbdCmd_Deg"
  nmodeTlaRhCmdDeg5/1 -> SimInputBusCreator/29  "EngineRhFuelCut"
  Gain17/1 -> SimInputBusCreator/21  "REFSI_FD_IN_nmodeFlapLhIBPosn_Deg"
  U-Tail Rudder/1 -> Subsystem10/1(In1), Subsystem6/1(In1)
  Gain19/1 -> SimInputBusCreator/25  "REFSI_FD_IN_nmodeFlapRhIBPosn_Deg"
  Gain16/1 -> SimInputBusCreator/20  "REFSI_FD_IN_nmodeFlapLhOBPosn_Deg"
  Subsystem1/1(CLAWS_AilLwrLhCmdDeg) -> SimInputBusCreator/2
  "WingletRudder "/1 -> Subsystem/1(In1), Subsystem16/1(In1)
  Subsystem3/1(CLAWS_ElvLhOBCmdDeg) -> SimInputBusCreator/4
  Subsystem7/1(CLAWS_ElvUTailLhCmdDeg) -> SimInputBusCreator/8
  Gain12/1 -> SimInputBusCreator/34  "REFSI_FD_IN_nmodeSplrRhInbdCmd_Deg"
  Subsystem15/1(CLAWS_AilLwrRhCmdDeg) -> SimInputBusCreator/16
  CG_Shifter/1 -> SimInputBusCreator/36  "REFSI_FD_IN_nmodeCgShifterKartPosCmd_Ft"
  Gain11/1 -> SimInputBusCreator/33  "REFSI_FD_IN_nmodeSplrLhInbdCmd_Deg"
  Brake/1 -> unity36/1, unity35/1, SimInputBusCreator/30  "REFSI_FD_IN_nmodeBrakeCmd"
  U-Tail Elevator/1 -> Subsystem9/1(In1), Subsystem7/1(In1)
  SimInputBusCreator/1 -> Command Bundle/1
  Gain/1 -> Subsystem14/1(In1)
  Gain1/1 -> Subsystem15/1(In1)
  Gain2/1 -> Subsystem12/1(In1)
  Gain3/1 -> Subsystem13/1(In1)
  Gain4/1 -> Subsystem1/1(In1)
  Gain5/1 -> Subsystem2/1(In1)
  Gain6/1 -> Subsystem3/1(In1)
  Gain7/1 -> Subsystem4/1(In1)
  Constant1/1 -> SimInputBusCreator/38  "pilotNzCmd_g"
  Constant/1 -> SimInputBusCreator/37  "piccoloInCmd"
  Constant2/1 -> SimInputBusCreator/39  "isControlSurfaceCmdFromSystem"
  Constant3/1 -> SimInputBusCreator/40  "nmodeReset"
  nmodeTlaRhCmdDeg4/1 -> SimInputBusCreator/41  "RefWindDirDeg"
  nmodeTlaRhCmdDeg6/1 -> SimInputBusCreator/42  "RefWindSpdKts"
  unity36/1 -> SimInputBusCreator/45  "PedalBrakeRh"
  unity35/1 -> SimInputBusCreator/44  "PedalBrakeLh"
  Gain8/1 -> SimInputBusCreator/26  "REFSI_FD_IN_nmodeTlaLhCmd_Deg"
  Gain9/1 -> SimInputBusCreator/27  "REFSI_FD_IN_nmodeTlaRhCmd_Deg"
  Aileron/1 -> Bus Selector/1
  Bus Selector/1 -> Gain4/1  "<PrtAileronUpperCmd_Deg>"
  Bus Selector/2 -> Gain5/1  "<PrtAileronLowerCmd_Deg>"
  Bus Selector/3 -> Gain/1  "<StbdAileronUpperCmd_Deg>"
  Bus Selector/4 -> Gain1/1  "<StbdAileronLowerCmd_Deg>"
  Outboard Elevon/1 -> Bus Selector1/1
  Bus Selector1/1 -> Gain6/1  "<PrtOutElevonCmd_Deg>"
  Bus Selector1/2 -> Gain3/1  "<StbdOutElevonCmd_Deg>"
  "Throttle "/1 -> Bus Selector2/1
  Bus Selector2/1 -> Gain8/1  "<PrtThrottleCmd_Pct>"
  Bus Selector2/2 -> Gain9/1  "<StbdThrottleCmd_Pct>"
  Inboard Elevon/1 -> Bus Selector3/1
  Bus Selector3/1 -> Gain7/1  "<PrtInbElevonCmd_Deg>"
  Bus Selector3/2 -> Gain2/1  "<StbdInbElevonCmd_Deg>"
  Spoilers/1 -> Gain13/1, Gain12/1, Gain11/1, Gain10/1
  Slats/1 -> Gain15/1, Gain14/1
  Flaps/1 -> Gain19/1, Gain18/1, Gain17/1, Gain16/1
  Constant4/1 -> SimInputBusCreator/46  "REFSI_FD_IN_nmodeCgShifterCmdType"
  Constant6/1 -> SimInputBusCreator/47  "REFSI_FD_IN_nmodeCgShifterNRCActive"

== system Lib_Piccolo/A//C Dynamics Full Interface/Simulated Piccolo Commands/7p ==
  Aileron : Inport
  Inboard Elevon : Inport  Port=2
  Outboard Elevon : Inport  Port=3
  U-Tail Elevator : Inport  Port=4
  Aft-Flap : Inport  Port=5
  "PylonRudder " : Inport  Port=6
  "WingletRudder " : Inport  Port=7
  U-Tail Rudder : Inport  Port=8
  "Throttle " : Inport  Port=9
  Nosegear : Inport  Port=10
  Flaps : Inport  Port=11
  Slats : Inport  Port=12
  Spoilers : Inport  Port=13
  Brake : Inport  Port=14
  Stabilizer : Inport  Port=15
  CG_Shifter : Inport  Port=16
  Add : Sum  Commented=on  Inputs=|++
  Bus Selector : BusSelector  OutputSignals=PrtAileronUpperCmd_Deg,PrtAileronLowerCmd_Deg,StbdAileronUpperCmd_Deg,StbdAileronLowerCmd_Deg
  Bus Selector1 : BusSelector  OutputSignals=PrtOutElevonCmd_Deg,StbdOutElevonCmd_Deg
  Bus Selector2 : BusSelector  OutputSignals=PrtThrottleCmd_Pct,StbdThrottleCmd_Pct
  Bus Selector3 : BusSelector  OutputSignals=PrtInbElevonCmd_Deg,StbdInbElevonCmd_Deg
  Constant : Constant  Value=0
  Constant1 : Constant  Value=0
  Constant2 : Constant  Value=0
  Constant3 : Constant
  Gain{,1..20} (21 alike) : Gain
  Goto Tag Visibility1 : GotoTagVisibility  GotoTag=CLAWsOn
  Signal Builder2 : Subsystem  Tag=STV Subsys  Commented=on  LoadFcn=sigbuilder_block('load');  StartFcn=sigbuilder_block('start');  StopFcn=sigbuilder_block('stop');  ClipboardFcn=sigbuilder_block('clipboard');  mask(Sigbuilder block){tuvar=[0:10]}
      mask help: Simulink:masks:SigbuilderBlock_MD
      mask init:
      | if ~strcmp(get_param(bdroot(gcbh),'SimulationStatus'),'stopped') tuvar = sigbuilder_block('maskInit'); end
      settings: CopyFcn=sigbuilder_block('copy');  DeleteFcn=sigbuilder_block('delete');  ModelCloseFcn=sigbuilder_block('modelClose');  PreSaveFcn=sigbuilder_block('preSave');  PauseFcn=sigbuilder_block('pause');  ContinueFcn=sigbuilder_block('continue');  NameChangeFcn=sigbuilder_block('namechange');  OpenFcn=sigbuilder_block('open',[421.8 380.4 544.2 313.2 ]);  CloseFcn=sigbuilder_block('close');
      mask Display: plot(0, 0, 100, 100,[2, 2, 32, 32, 2], [68, 8, 8, 68, 68],[32, 2], [38, 38], [32, 19, 2],[53, 60, 44], [32, 17, 17, 2],[16, 16, 31, 31]);txt = getActiveGroup(gcbh);text(2, 100, txt,'verticalAlignment', 'top');
  SimInputBusCreator : BusCreator  Inputs=43
  Subsystem : Subsystem
  Subsystem1 : Subsystem
  Subsystem10 : Subsystem
  Subsystem11 : Subsystem
  Subsystem12 : Subsystem
  Subsystem13 : Subsystem
  Subsystem14 : Subsystem
  Subsystem15 : Subsystem
  Subsystem16 : Subsystem
  Subsystem2 : Subsystem
  Subsystem3 : Subsystem
  Subsystem4 : Subsystem
  Subsystem5 : Subsystem
  Subsystem6 : Subsystem
  Subsystem7 : Subsystem
  Subsystem8 : Subsystem
  Subsystem9 : Subsystem
  Terminator : Terminator
  nmodeTlaRhCmdDeg1 : Constant  Commented=on  Value=Trim_piccoloInCmd
  nmodeTlaRhCmdDeg2 : Constant  Value=0
  nmodeTlaRhCmdDeg3 : Constant  Value=EngineLhFuelCut
  nmodeTlaRhCmdDeg4 : Constant  Value=WindDir_Deg
  nmodeTlaRhCmdDeg5 : Constant  Value=EngineRhFuelCut
  nmodeTlaRhCmdDeg6 : Constant  Value=WindSpd_Kts
  nmodeTlaRhCmdDeg7 : Constant  Value=WindVertSpd_Kts
  unity35 : Gain
  unity36 : Gain
  Command Bundle : Outport
  tag scope: CLAWsOn=scoped
  wires:
  nmodeTlaRhCmdDeg7/1 -> SimInputBusCreator/41  "VertWindSpdKts"
  Gain20/1 -> SimInputBusCreator/18  "REFSI_FD_IN_nmodeStabCmd"
  Subsystem4/1(CLAWS_ElvLhIBCmdDeg) -> SimInputBusCreator/5
  Subsystem/1(CLAWS_RudWingletLhCmdDeg) -> SimInputBusCreator/1
  nmodeTlaRhCmdDeg3/1 -> SimInputBusCreator/27  "EngineLhFuelCut"
  Subsystem2/1(CLAWS_AilUprLhCmdDeg) -> SimInputBusCreator/3
  Gain15/1 -> SimInputBusCreator/22  "REFSI_FD_IN_nmodeSlatRhPosn_Deg"
  Gain14/1 -> SimInputBusCreator/21  "REFSI_FD_IN_nmodeSlatLhPosn_Deg"
  Subsystem10/1(CLAWS_RudUTailRhCmdDeg) -> SimInputBusCreator/11
  Subsystem14/1(CLAWS_AilUprRhCmdDeg) -> SimInputBusCreator/15
  Subsystem6/1(CLAWS_RudUTailLhCmdDeg) -> SimInputBusCreator/7
  Subsystem5/1(CLAWS_RudPylLhCmdDeg) -> SimInputBusCreator/6
  Subsystem8/1(CLAWS_AftFlapCmdDeg) -> SimInputBusCreator/9
  Nosegear/1 -> SimInputBusCreator/30  "REFSI_FD_IN_nmodeNoseGearCmd_Deg"
  Subsystem12/1(CLAWS_ElvRhIBCmdDeg) -> SimInputBusCreator/13
  Subsystem16/1(CLAWS_RudWingletRhCmdDeg) -> SimInputBusCreator/17
  Gain10/1 -> SimInputBusCreator/31  "REFSI_FD_IN_nmodeSplrLhOutbdCmd_Deg"
  nmodeTlaRhCmdDeg2/1 -> [CLAWsOn]
  Subsystem13/1(CLAWS_ElvRhOBCmdDeg) -> SimInputBusCreator/14
  Aft-Flap/1 -> Subsystem8/1(In1)
  Signal Builder2/1(Signal 3) -> Add/2
  nmodeTlaRhCmdDeg1/1 -> Add/1
  Subsystem11/1(CLAWS_RudPylRhCmdDeg) -> SimInputBusCreator/12
  "PylonRudder "/1 -> Subsystem11/1(In1), Subsystem5/1(In1)
  Gain18/1 -> SimInputBusCreator/23  "REFSI_FD_IN_nmodeFlapRhOBPosn_Deg"
  Subsystem9/1(CLAWS_ElvUTailRhCmdDeg) -> SimInputBusCreator/10
  Gain13/1 -> SimInputBusCreator/34  "REFSI_FD_IN_nmodeSplrRhOutbdCmd_Deg"
  nmodeTlaRhCmdDeg5/1 -> SimInputBusCreator/28  "EngineRhFuelCut"
  Gain17/1 -> SimInputBusCreator/20  "REFSI_FD_IN_nmodeFlapLhIBPosn_Deg"
  U-Tail Rudder/1 -> Subsystem10/1(In1), Subsystem6/1(In1)
  Gain19/1 -> SimInputBusCreator/24  "REFSI_FD_IN_nmodeFlapRhIBPosn_Deg"
  Gain16/1 -> SimInputBusCreator/19  "REFSI_FD_IN_nmodeFlapLhOBPosn_Deg"
  Subsystem1/1(CLAWS_AilLwrLhCmdDeg) -> SimInputBusCreator/2
  "WingletRudder "/1 -> Subsystem/1(In1), Subsystem16/1(In1)
  Subsystem3/1(CLAWS_ElvLhOBCmdDeg) -> SimInputBusCreator/4
  Subsystem7/1(CLAWS_ElvUTailLhCmdDeg) -> SimInputBusCreator/8
  Gain12/1 -> SimInputBusCreator/33  "REFSI_FD_IN_nmodeSplrRhInbdCmd_Deg"
  Subsystem15/1(CLAWS_AilLwrRhCmdDeg) -> SimInputBusCreator/16
  CG_Shifter/1 -> Terminator/1  "REFSI_FD_IN_nmodeCgShifterCmd_Ft"
  Gain11/1 -> SimInputBusCreator/32  "REFSI_FD_IN_nmodeSplrLhInbdCmd_Deg"
  Brake/1 -> unity36/1, unity35/1, SimInputBusCreator/29  "REFSI_FD_IN_nmodeBrakeCmd"
  U-Tail Elevator/1 -> Subsystem9/1(In1), Subsystem7/1(In1)
  SimInputBusCreator/1 -> Command Bundle/1
  Gain/1 -> Subsystem14/1(In1)
  Gain1/1 -> Subsystem15/1(In1)
  Gain2/1 -> Subsystem12/1(In1)
  Gain3/1 -> Subsystem13/1(In1)
  Gain4/1 -> Subsystem1/1(In1)
  Gain5/1 -> Subsystem2/1(In1)
  Gain6/1 -> Subsystem3/1(In1)
  Gain7/1 -> Subsystem4/1(In1)
  Constant1/1 -> SimInputBusCreator/36  "pilotNzCmd_g"
  Constant/1 -> SimInputBusCreator/35  "piccoloInCmd"
  Constant2/1 -> SimInputBusCreator/37  "isControlSurfaceCmdFromSystem"
  Constant3/1 -> SimInputBusCreator/38  "nmodeReset"
  nmodeTlaRhCmdDeg4/1 -> SimInputBusCreator/39  "RefWindDirDeg"
  nmodeTlaRhCmdDeg6/1 -> SimInputBusCreator/40  "RefWindSpdKts"
  unity36/1 -> SimInputBusCreator/43  "PedalBrakeRh"
  unity35/1 -> SimInputBusCreator/42  "PedalBrakeLh"
  Gain8/1 -> SimInputBusCreator/25  "REFSI_FD_IN_nmodeTlaLhCmd_Deg"
  Gain9/1 -> SimInputBusCreator/26  "REFSI_FD_IN_nmodeTlaRhCmd_Deg"
  Aileron/1 -> Bus Selector/1
  Bus Selector/1 -> Gain4/1  "<PrtAileronUpperCmd_Deg>"
  Bus Selector/2 -> Gain5/1  "<PrtAileronLowerCmd_Deg>"
  Bus Selector/3 -> Gain/1  "<StbdAileronUpperCmd_Deg>"
  Bus Selector/4 -> Gain1/1  "<StbdAileronLowerCmd_Deg>"
  Outboard Elevon/1 -> Bus Selector1/1
  Bus Selector1/1 -> Gain6/1  "<PrtOutElevonCmd_Deg>"
  Bus Selector1/2 -> Gain3/1  "<StbdOutElevonCmd_Deg>"
  "Throttle "/1 -> Bus Selector2/1
  Bus Selector2/1 -> Gain8/1  "<PrtThrottleCmd_Pct>"
  Bus Selector2/2 -> Gain9/1  "<StbdThrottleCmd_Pct>"
  Inboard Elevon/1 -> Bus Selector3/1
  Bus Selector3/1 -> Gain7/1  "<PrtInbElevonCmd_Deg>"
  Bus Selector3/2 -> Gain2/1  "<StbdInbElevonCmd_Deg>"
  Spoilers/1 -> Gain13/1, Gain12/1, Gain11/1, Gain10/1
  Slats/1 -> Gain15/1, Gain14/1
  Flaps/1 -> Gain19/1, Gain18/1, Gain17/1, Gain16/1
  Stabilizer/1 -> Gain20/1

== system Lib_Piccolo/Airspeed Complementary Filter/HPF Acceleration/LFP Nx ==
  Input : Inport
  Reset : Inport  Port=2
  Add1 : Sum  Inputs=++|
  Compare To Constant2 : simulink/Logic and Bit Operations/Compare To Constant  relop=>  const=0  OutDataTypeStr=uint8
  Constant11 : Constant  Value=TasLpfCutoff
  Switch1 : Switch  Criteria=u2 > Threshold
  Unit Delay1 : UnitDelay  InitialCondition=LPFtasInit  SampleTime=-1
  a1 : Gain  Gain=1-Fp_TAS_Filter
  b0 : Gain  Gain=Fp_TAS_Filter
  Output : Outport
  wires:
  Unit Delay1/1 -> a1/1
  b0/1 -> Add1/2
  a1/1 -> Add1/1
  Add1/1 -> Unit Delay1/1, Switch1/1
  Input/1 -> Switch1/3, b0/1
  Switch1/1 -> Output/1
  Compare To Constant2/1 -> Switch1/2
  Constant11/1 -> Compare To Constant2/1
